simulink model "UDPtest"  (R2025b)
settings: Solver=FixedStepDiscrete  StartTime=0.0  StopTime=10.0  FixedStep=0.04  RelTol=1e-3
settings Model: Creator=Administrator  LastModifiedBy=Administrator

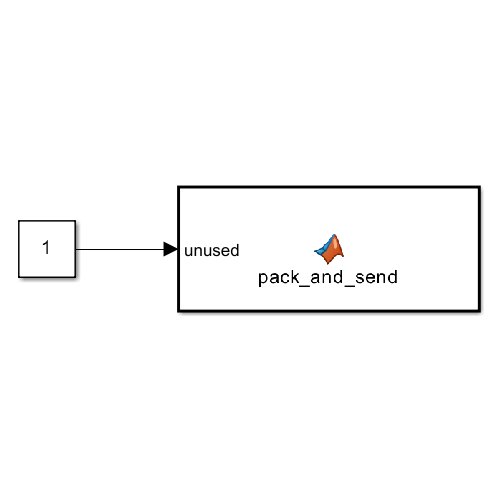
[thumbnail: Simulink's stored preview of the top-level diagram]
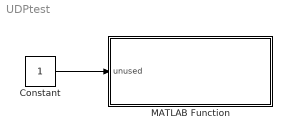
== system UDPtest ==
  Constant : Constant
  MATLAB Function : MATLAB Function  TreatAsAtomicUnit=on
  wires:
  Constant/1 -> MATLAB Function/1(unused)

== matlab function UDPtest/MATLAB Function ==
  data: unused input
function pack_and_send(~)   %#codegen
% 固定包测试：每步发一帧，seq 自增

persistent u seq_num;
coder.extrinsic('udpport', 'write');   % 告诉代码生成器这些是外部函数

if isempty(u)
  u       = udpport("byte", "LocalPort", 12345);
  seq_num = uint32(0);
end

seq_num = seq_num + uint32(1);

pkt = [typecast(seq_num,      'uint8'), ...
     typecast(single( 10.5),  'uint8'), ...
     typecast(single( 20.5),  'uint8'), ...
     typecast(single( 30.5),  'uint8'), ...
     typecast(single(  1.5),  'uint8'), ...
     typecast(single(  2.5),  'uint8'), ...
     typecast(single(  3.5),  'uint8')];

write(u, pkt, "uint8", "192.168.1.100", 8080);
